simulink model "Brightspace_model"  (R2020b)
settings: Solver=VariableStepAuto  StartTime=0.0  StopTime=5  RelTol=1e-3
libraries: pid_lib x2
settings Model: Creator=Simon Gebraad  LastModifiedBy=Simon Gebraad

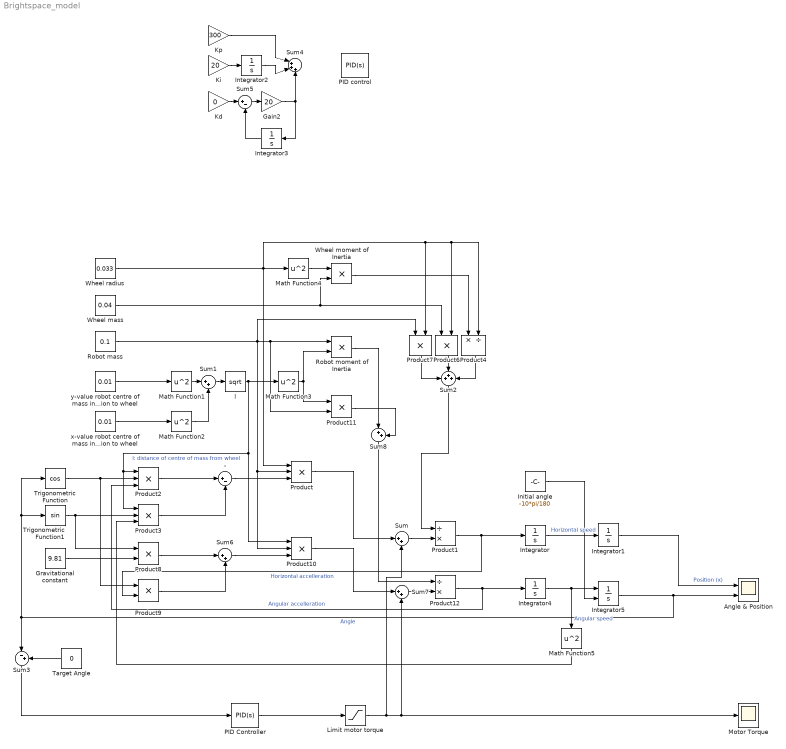
== system Brightspace_model ==
  - : Sum  Inputs=|+-
  Angle & Position : Scope  NumInputPorts=2
  Gain2 : Gain  Gain=20
  Gravitational constant : Constant  Value=9.81
  Initial angle : Constant  Value=-10*pi/180
  Integrator{,1..4} (5 alike) : Integrator
  Integrator5 : Integrator  InitialConditionSource=external  InitialCondition=1
  Kd : Gain  Gain=0
  Ki : Gain  Gain=20
  Kp : Gain  Gain=300
  Limit motor torque : Saturate
  Math Function{1..5} (5 alike) : Math  Operator=square  SaturateOnIntegerOverflow=on
  Motor Torque : Scope
  PID Controller : pid_lib/PID Controller  Controller=PID  Form=Parallel  TimeDomain=Continuous-time  UseExternalTs=off  SampleTime=-1  IntegratorMethod=Forward Euler  FilterMethod=Forward Euler  ControllerParametersSource=internal  P=0.169458425420138  I=1.35754870528882  D=0.000939082915534522  UseFilter=on  N=10073.1070418419  TunerSelectOption=Transfer Function Based (PID Tuner App)  InitialConditionSource=internal  InitialConditionForIntegrator=0  InitialConditionForFilter=0  DifferentiatorICPrevScaledInput=0  ExternalReset=none  TrackingMode=off  Kt=1  LimitOutput=off  SatLimitsSource=internal  UpperSaturationLimit=inf  LowerSaturationLimit=-inf  LinearizeAsGain=on  AntiWindupMode=none  Kb=1  POutMin=[]  POutMax=[]  IOutMin=[]  IOutMax=[]  DOutMin=[]  DOutMax=[]  NOutMin=[]  NOutMax=[]  SumOutMin=[]  SumOutMax=[]  SaturationOutMin=[]  SaturationOutMax=[]  PParamMin=[]  PParamMax=[]  IParamMin=[]  IParamMax=[]  DParamMin=[]  DParamMax=[]  NParamMin=[]  NParamMax=[]  KbParamMin=[]  KbParamMax=[]  KtParamMin=[]  KtParamMax=[]  KbOutMin=[]  KbOutMax=[]  KtOutMin=[]  KtOutMax=[]  IntegratorOutMin=[]  IntegratorOutMax=[]  FilterOutMin=[]  FilterOutMax=[]  SumI1OutMin=[]  SumI1OutMax=[]  SumI2OutMin=[]  SumI2OutMax=[]  SumI3OutMin=[]  SumI3OutMax=[]  SumI4OutMin=[]  SumI4OutMax=[]  SumDOutMin=[]  SumDOutMax=[]  DifferentiatorOutMin=[]  DifferentiatorOutMax=[]  FilterDiffOutCoefMin=[]  FilterDiffOutCoefMax=[]  ReciprocalOutMin=[]  ReciprocalOutMax=[]  SumDenOutMin=[]  SumDenOutMax=[]  SumNumOutMin=[]  SumNumOutMax=[]  DivideOutMin=[]  DivideOutMax=[]  UdiffTsProdOutMin=[]  UdiffTsProdOutMax=[]  NTsProdOutMin=[]  NTsProdOutMax=[]  UintegralTsProdOutMin=[]  UintegralTsProdOutMax=[]  UngainTsProdOutMin=[]  UngainTsProdOutMax=[]  IntegratorContinuousStateAttributes=''  IntegratorStateMustResolveToSignalObject=off  IntegratorRTWStateStorageClass=Auto  FilterContinuousStateAttributes=''  FilterStateMustResolveToSignalObject=off  FilterRTWStateStorageClass=Auto  ParallelPVariant=InternalParameters  IdealPVariant=Disabled  IVariant=InternalParameters  DVariant=InternalParameters  IntegratorVariant=Continuous  SatVariant=Disabled  AWVariant=Passthrough  PCopyVariant=Disabled  TRVariant=Disabled  FdbkBlocksVariant=Forward  IdealPFdbkVariant=Disabled  SatFdbkVariant=Disabled  DerivativeFilterVariant=ContFilter  NVariant=InternalParameters  NCopyVariant=Disabled  FilterICVariant=InternalICsFilter  IntegratorICVariant=InternalICs  ExternalResetVariant=Disabled  TRSumVariant=Passthrough  SumFdbkVariant=Disabled  SumVariant=Sum_PID  TsampFilterVariant=InternalTs  TsampNgainVariant=Passthrough  TsampIntegralVariant=Passthrough  ExternalSaturationOutDataTypeStr=Inherit: Same as second input
  PID control : pid_lib/PID Controller  Controller=PID  Form=Parallel  TimeDomain=Continuous-time  UseExternalTs=off  SampleTime=-1  IntegratorMethod=Forward Euler  FilterMethod=Forward Euler  ControllerParametersSource=internal  P=3.60881190211891  I=34.4753313656519  D=0.0933922260980466  UseFilter=on  N=20796.0504924641  TunerSelectOption=Transfer Function Based (PID Tuner App)  InitialConditionSource=internal  InitialConditionForIntegrator=0  InitialConditionForFilter=0  DifferentiatorICPrevScaledInput=0  ExternalReset=none  TrackingMode=off  Kt=1  LimitOutput=off  SatLimitsSource=internal  UpperSaturationLimit=inf  LowerSaturationLimit=-inf  LinearizeAsGain=on  AntiWindupMode=none  Kb=1  POutMin=[]  POutMax=[]  IOutMin=[]  IOutMax=[]  DOutMin=[]  DOutMax=[]  NOutMin=[]  NOutMax=[]  SumOutMin=[]  SumOutMax=[]  SaturationOutMin=[]  SaturationOutMax=[]  PParamMin=[]  PParamMax=[]  IParamMin=[]  IParamMax=[]  DParamMin=[]  DParamMax=[]  NParamMin=[]  NParamMax=[]  KbParamMin=[]  KbParamMax=[]  KtParamMin=[]  KtParamMax=[]  KbOutMin=[]  KbOutMax=[]  KtOutMin=[]  KtOutMax=[]  IntegratorOutMin=[]  IntegratorOutMax=[]  FilterOutMin=[]  FilterOutMax=[]  SumI1OutMin=[]  SumI1OutMax=[]  SumI2OutMin=[]  SumI2OutMax=[]  SumI3OutMin=[]  SumI3OutMax=[]  SumI4OutMin=[]  SumI4OutMax=[]  SumDOutMin=[]  SumDOutMax=[]  DifferentiatorOutMin=[]  DifferentiatorOutMax=[]  FilterDiffOutCoefMin=[]  FilterDiffOutCoefMax=[]  ReciprocalOutMin=[]  ReciprocalOutMax=[]  SumDenOutMin=[]  SumDenOutMax=[]  SumNumOutMin=[]  SumNumOutMax=[]  DivideOutMin=[]  DivideOutMax=[]  UdiffTsProdOutMin=[]  UdiffTsProdOutMax=[]  NTsProdOutMin=[]  NTsProdOutMax=[]  UintegralTsProdOutMin=[]  UintegralTsProdOutMax=[]  UngainTsProdOutMin=[]  UngainTsProdOutMax=[]  IntegratorContinuousStateAttributes=''  IntegratorStateMustResolveToSignalObject=off  IntegratorRTWStateStorageClass=Auto  FilterContinuousStateAttributes=''  FilterStateMustResolveToSignalObject=off  FilterRTWStateStorageClass=Auto  ParallelPVariant=InternalParameters  IdealPVariant=Disabled  IVariant=InternalParameters  DVariant=InternalParameters  IntegratorVariant=Continuous  SatVariant=Disabled  AWVariant=Passthrough  PCopyVariant=Disabled  TRVariant=Disabled  FdbkBlocksVariant=Forward  IdealPFdbkVariant=Disabled  SatFdbkVariant=Disabled  DerivativeFilterVariant=ContFilter  NVariant=InternalParameters  NCopyVariant=Disabled  FilterICVariant=InternalICsFilter  IntegratorICVariant=InternalICs  ExternalResetVariant=Disabled  TRSumVariant=Passthrough  SumFdbkVariant=Disabled  SumVariant=Sum_PID  TsampFilterVariant=InternalTs  TsampNgainVariant=Passthrough  TsampIntegralVariant=Passthrough  ExternalSaturationOutDataTypeStr=Inherit: Same as second input
  Product{,2..3,10} (4 alike) : Product  Inputs=3
  Product1 : Product  Inputs=/*
  Product{6..9,11} (5 alike) : Product
  Product12 : Product  Inputs=/*
  Product4 : Product  Inputs=*/
  Robot mass : Constant  Value=0.1
  Robot moment of Inertia : Product
  Sum{,1,6..8} (5 alike) : Sum  Inputs=|++
  Sum2 : Sum  Inputs=+++
  Sum3 : Sum  Inputs=|-+
  Sum4 : Sum  Inputs=|+++
  Sum5 : Sum  Inputs=|+-
  Target Angle : Constant  Value=0
  Trigonometric Function : Trigonometry  Operator=cos
  Trigonometric Function1 : Trigonometry
  Wheel mass : Constant  Value=0.04
  Wheel moment of Inertia : Product
  Wheel radius : Constant  Value=0.033
  l : Sqrt  SaturateOnIntegerOverflow=on
  x-value robot centre of mass in relation to wheel : Constant  Value=0.01
  y-value robot centre of mass in relation to wheel : Constant  Value=0.01
  wires:
  Robot mass/1 -> Product7/1, Product10/2, Product/2, Robot moment of Inertia/1, Product11/2
  Product/1 -> Sum/1
  Sum/1 -> Product1/2
  Integrator/1 -> Integrator1/1  "Horizontal speed"
  Integrator1/1 -> Angle & Position/1  "Position (x)"
  Ki/1 -> Integrator2/1
  Kp/1 -> Sum4/1
  Integrator2/1 -> Sum4/2
  Kd/1 -> Sum5/1
  Sum5/1 -> Gain2/1
  Gain2/1 -> Integrator3/1, Sum4/3
  Integrator3/1 -> Sum5/2
  Trigonometric Function/1 -> Product9/1, Product2/2
  x-value robot centre of mass in relation to wheel/1 -> Math Function2/1
  Trigonometric Function1/1 -> Product8/1, Product3/2
  Product2/1 -> -/1
  Product3/1 -> -/2
  -/1 -> Product/3
  y-value robot centre of mass in relation to wheel/1 -> Math Function1/1
  Math Function1/1 -> Sum1/1
  Math Function2/1 -> Sum1/2
  Sum1/1 -> l/1
  l/1 -> Product10/1, Product3/1, Product2/1, Math Function3/1  "l: distance of centre of mass from wheel"
  Math Function3/1 -> Product11/1, Robot moment of Inertia/2
  Product1/1 -> Product9/2, Integrator/1  "Horizontal accelleration"
  Wheel radius/1 -> Math Function4/1, Product7/2, Product4/2, Product6/2, Product/1
  Wheel mass/1 -> Product6/1, Wheel moment of Inertia/2
  Math Function4/1 -> Wheel moment of Inertia/1
  Wheel moment of Inertia/1 -> Product4/1
  Product7/1 -> Sum2/1
  Product6/1 -> Sum2/2
  Product4/1 -> Sum2/3
  Sum2/1 -> Product1/1
  Gravitational constant/1 -> Product8/2
  Product8/1 -> Sum6/1
  Product9/1 -> Sum6/2
  Sum6/1 -> Product10/3
  Product10/1 -> Sum7/1
  Robot moment of Inertia/1 -> Sum8/1
  Product11/1 -> Sum8/2
  Sum7/1 -> Product12/2
  Sum8/1 -> Product12/1
  Product12/1 -> Product2/3, Integrator4/1  "Angular accelleration"
  Integrator4/1 -> Math Function5/1, Integrator5/1  "Angular speed"
  Integrator5/1 -> Angle & Position/2, Sum3/1, Trigonometric Function/1, Trigonometric Function1/1  "Angle"
  Math Function5/1 -> Product3/3
  Target Angle/1 -> Sum3/2
  Initial angle/1 -> Integrator5/2
  Limit motor torque/1 -> Motor Torque/1, Sum7/2, Sum/2
  PID Controller/1 -> Limit motor torque/1
  Sum3/1 -> PID Controller/1
